simulink model "pfd1"  (R2024b)
settings: Solver=FixedStepAuto  StartTime=0.0  StopTime=10.0  FixedStep=Ts  RelTol=1e-3
settings Model: Creator=marti  LastModifiedBy=marti

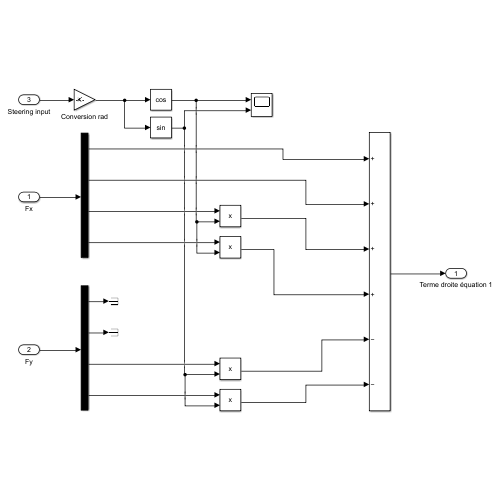
[thumbnail: Simulink's stored preview of the top-level diagram]
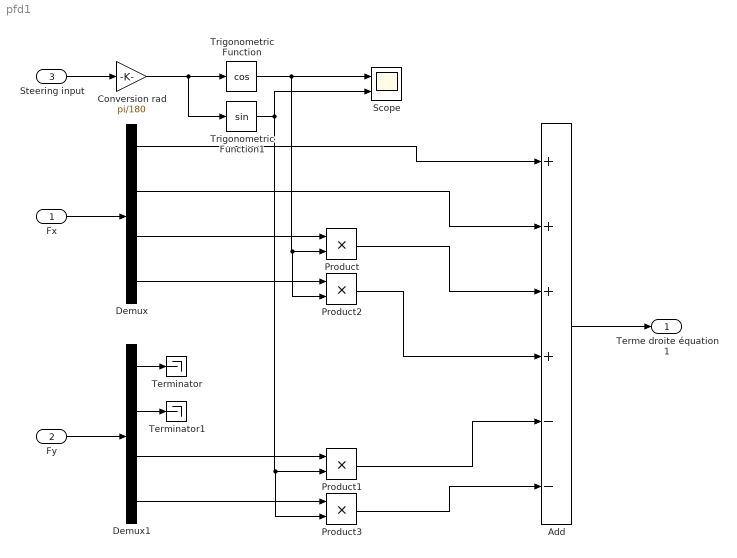
== system pfd1 ==
  Fx : Inport
  Fy : Inport  Port=2
  Steering input : Inport  Port=3
  Add : Sum  Inputs=++++--
  Conversion rad : Gain  Gain=pi/180
  Demux : Demux
  Demux1 : Demux
  Product{,1..3} (4 alike) : Product
  Scope : Scope  NumInputPorts=2
  Terminator : Terminator
  Terminator1 : Terminator
  Trigonometric Function : Trigonometry  Operator=cos
  Trigonometric Function1 : Trigonometry
  Terme droite équation 1 : Outport
  wires:
  Fx/1 -> Demux/1
  Fy/1 -> Demux1/1
  Steering input/1 -> Conversion rad/1
  Conversion rad/1 -> Trigonometric Function1/1, Trigonometric Function/1
  Demux/3 -> Product/1
  Demux/4 -> Product2/1
  Demux1/3 -> Product1/1
  Demux1/4 -> Product3/1
  Trigonometric Function/1 -> Scope/1, Product2/2, Product/2
  Trigonometric Function1/1 -> Scope/2, Product3/2, Product1/2
  Demux/1 -> Add/1
  Demux/2 -> Add/2
  Product/1 -> Add/3
  Product2/1 -> Add/4
  Product1/1 -> Add/5
  Product3/1 -> Add/6
  Add/1 -> Terme droite équation 1/1
  Demux1/1 -> Terminator/1
  Demux1/2 -> Terminator1/1
